simulink model "ex5"  (R2023b)
settings: Solver=VariableStepAuto  StartTime=0.0  StopTime=200  RelTol=1e-3
undefined symbols (not defined in the file): k
settings Model: Creator=Bianca  LastModifiedBy=Bianca

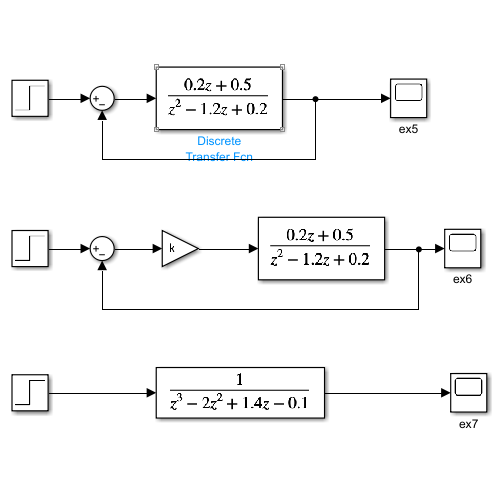
[thumbnail: Simulink's stored preview of the top-level diagram]
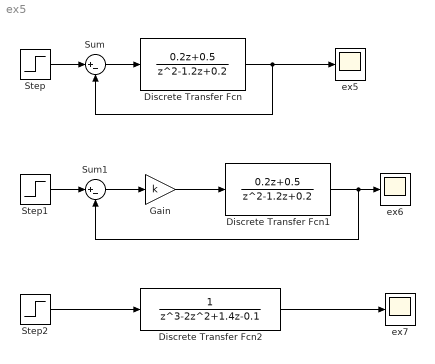
== system ex5 ==
  Discrete Transfer Fcn : DiscreteTransferFcn  Numerator=[0 0.2 0.5]  Denominator=[1 -1.2 0.2]  SampleTime=0.05
  Discrete Transfer Fcn1 : DiscreteTransferFcn  Numerator=[0 0.2 0.5]  Denominator=[1 -1.2 0.2]  SampleTime=0.05
  Discrete Transfer Fcn2 : DiscreteTransferFcn  Denominator=[1 -2 1.4 -0.1]  SampleTime=0.05
  Gain : Gain  Gain=k
  Step : Step  After=5  SampleTime=0
  Step1 : Step  After=5  SampleTime=0
  Step2 : Step  Time=10  After=8  SampleTime=0
  Sum : Sum  Inputs=|+-
  Sum1 : Sum  Inputs=|+-
  ex5 : Scope
  ex6 : Scope
  ex7 : Scope
  wires:
  Discrete Transfer Fcn/1 -> Sum/2, ex5/1
  Step/1 -> Sum/1
  Sum/1 -> Discrete Transfer Fcn/1
  Step1/1 -> Sum1/1
  Discrete Transfer Fcn1/1 -> Sum1/2, ex6/1
  Sum1/1 -> Gain/1
  Gain/1 -> Discrete Transfer Fcn1/1
  Discrete Transfer Fcn2/1 -> ex7/1
  Step2/1 -> Discrete Transfer Fcn2/1
